simulink model "Week2Problem4"  (R2020b)
settings: Solver=VariableStepAuto  StartTime=0.0  StopTime=10.0  RelTol=1e-3
values from neighbouring files (symbols this model uses):
  Kd = 0.04    [Parameter.m]
  Ki = 51    [Parameter.m]
  Kp = 5    [Parameter.m]
settings Model: DataDictionary=problem4.sldd  Creator=HP  LastModifiedBy=HP

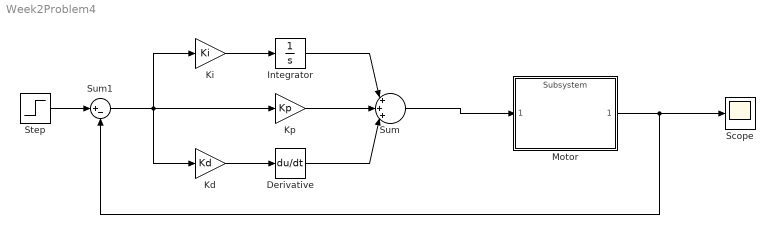
== system Week2Problem4 ==
  Derivative : Derivative
  Integrator : Integrator
  Kd : Gain  Gain=Kd
  Ki : Gain  Gain=Ki
  Kp : Gain  Gain=Kp
  Motor : ModelReference  ModelNameDialog=Subsystem  SimulationMode=Normal  ModelReferenceVersion=1.8
  Scope : Scope
  Step : Step  SampleTime=0
  Sum : Sum  Inputs=|+++|
  Sum1 : Sum  Inputs=|+-
  wires:
  Kp/1 -> Sum/2
  Motor/1 -> Scope/1, Sum1/2
  Sum/1 -> Motor/1
  Sum1/1 -> Ki/1, Kd/1, Kp/1
  Ki/1 -> Integrator/1
  Integrator/1 -> Sum/1
  Derivative/1 -> Sum/3
  Kd/1 -> Derivative/1
  Step/1 -> Sum1/1
